simulink model "PubIfDecisionTOS_MDL"  (R2020b)
settings: configuration reference "DspaceConfig" (kept outside this file)
PostLoadFcn:
  | if any(exist('dsrtsu_mdlpostloadfcn', 'file') ~= 0), dsrtsu_mdlpostloadfcn('Execute', bdroot); end
InitFcn:
  | , if any(exist('dsmpb_private', 'file') ~= 0), dsmpb_private('dsmpb_mdlclblib', 'Init', bdroot); end,
undefined symbols (not defined in the file or in its folder): C_TOS_ACCEgoRAxletoFbumplength_m, C_TOS_ACCTargetFront_Flag, C_TOS_AEBJAPedObjDxThre_Val, C_TOS_AEBJAPedObjDyThre_Val, C_TOS_AEBJATargetSize_Val, C_TOS_AEBJAVehObjDxThre_Val, C_TOS_AEBJAVehObjDyThre_Val, C_TOS_AEBJuncPedTargetSize_Val, C_TOS_AEBLatObjDxThre_Val, C_TOS_AEBLatPedDyThre_Val, C_TOS_AEBLatTargetSize_Val, C_TOS_AEBLongTargetInEgoFront_Flag, C_TOS_axAbsGround_Parameter, C_TOS_CameraConfirmedFlag, C_TOS_CNsubjWidth, C_TOS_CurrentLaneCoreMinWidth_Val, C_TOS_CutInProb_Val_Zero, C_TOS_CutOutProb_Val_Zero, C_TOS_D2R_Val, C_TOS_DefaultValueObjectToCenterLine_dy, C_TOS_EgoCarWidth_Val, C_TOS_EgoDxRefPoint_m, C_TOS_EgoRAxletoFbumplength_m, C_TOS_HalfWidthVehicle_Con, C_TOS_HWA_CurrentLaneFlag, C_TOS_HWA_LeftLaneFlag, C_TOS_HWA_MovingDir_Vaild, C_TOS_HWA_MovState_Vaild, C_TOS_HWA_RightLaneFlag, C_TOS_LaneLineCourseErrorFront, C_TOS_LaneLineCourseErrorRear, C_TOS_MotorbikeDefaultWidth_m, C_TOS_NumberOfEffectiveTargets, C_TOS_Obj_Age_Val, C_TOS_Objdx_Constraint_Val, C_TOS_ObjectDefaultWidth_m, C_TOS_ObjInCurrentLane_Val, C_TOS_ObjInCurrentLaneValid, C_TOS_ObjInLeftLaneValid, C_TOS_ObjInRightLaneValid, C_TOS_ObjNotInCurrentLane_Val, C_TOS_ObjNotREElementType, C_TOS_ObjPredictDis_dy_ConstantVal_Zeros, C_TOS_ObjToCenterLine_ConstantVal_Zeros, C_TOS_OFMObjIDInvilad_Val, C_TOS_PIL_LatDisCons_Val_zero, C_TOS_PIL_ObjectCutInFlag_b, C_TOS_PIL_ObjectCutOutFlag_b, C_TOS_PIL_ObjLaneProb_al_Val, C_TOS_PP_ObjFusType_FC_Confirm_b, C_TOS_PP_ObjFusType_FC_FR_Confirm_b, C_TOS_PP_ObjFusType_FR_Confirm_b, C_TOS_RE_80BoolDefault_Val, C_TOS_RE_80Single181Default_Val, C_TOS_RE_80Single255Default_Val, C_TOS_RE_80Uint8Default_Val, C_TOS_RE_D2R, C_TOS_RE_D_180_Val, C_TOS_RE_InvalidObjectID_Val, C_TOS_RE_InvalidTargetChainDir_Val ... (+142)
libraries: simulink x1650, TOS_LIB x361, canfdmsglib x14
(part 54 of 69)

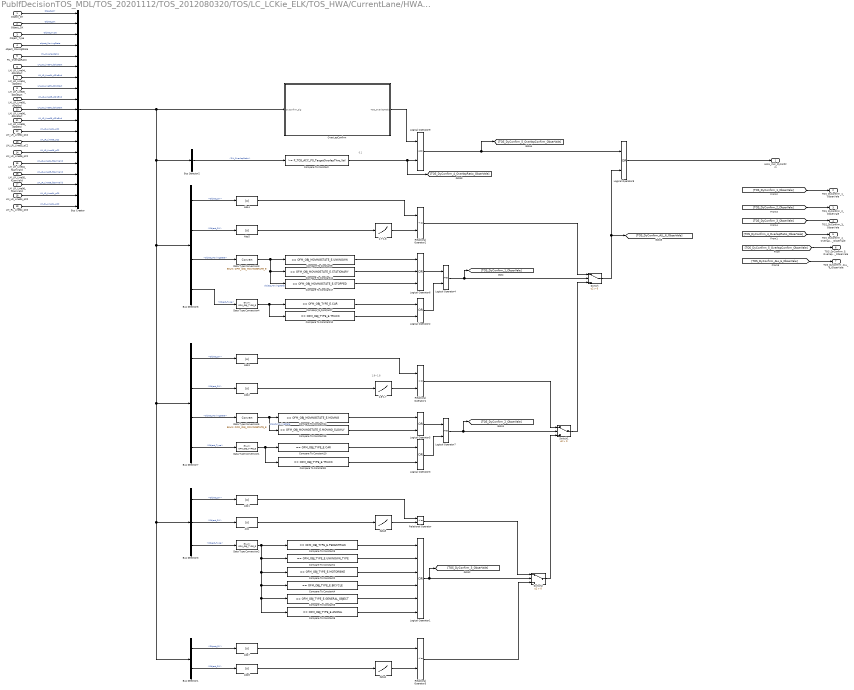
== system PubIfDecisionTOS_MDL/TOS_20201112/TOS_2012080320/TOS/LC_LCKie_ELK/TOS_HWA/CurrentLane/HWA_CurrentLane_Target/HWA_CLF_Target_1/HWA_CLF_Target/HWA_CLF_Target/HWA_CLF_DyConfirm ==
  note: 0.1
  note: 1.9~1.8
  Object_DY : Inport
  Object_DX : Inport  Port=2
  Object_Type : Inport  Port=3
  object_MovingState : Inport  Port=4
  PIL_OverlapRatio : Inport  Port=5
  LM_LR_Line04_dDisStart : Inport  Port=6
  LM_LR_Line04_dDisEnd : Inport  Port=7
  LM_LR_Line05_dDisStart : Inport  Port=8
  LM_LR_Line05_dDisEnd : Inport  Port=9
  LM_LR_Line06_dDisStart : Inport  Port=10
  LM_LR_Line06_dDisEnd : Inport  Port=11
  LM_LR_Line04_pC2 : Inport  Port=12
  LM_LR_Line05_pC2 : Inport  Port=13
  LM_LR_Line06_pC2 : Inport  Port=14
  LM_LR_Line04_fCamValid : Inport  Port=15
  LM_LR_Line05_fCamValid : Inport  Port=16
  LM_LR_Line06_fCamValid : Inport  Port=17
  LM_LR_Line04_pC0 : Inport  Port=18
  LM_RL_Line04_pC0 : Inport  Port=19
  1.7-1.6 : Lookup_n-D  NumberOfTableDimensions=1  BreakpointsForDimension1=[0,20,40,60,80,100,120,140]  Table=[1.7,1.7,1.65,1.65,1.6,1.6,1.6,1.6]  RndMeth=Simplest  InputSameDT=on
  1.8-1.7 : Lookup_n-D  NumberOfTableDimensions=1  BreakpointsForDimension1=[0,20,40,60,80,100,120,140]  Table=[1.8,1.8,1.75,1.75,1.7,1.7,1.7,1.7]  RndMeth=Simplest  InputSameDT=on
  Abs{,1..7} (8 alike) : Abs
  Bus Creator : BusCreator  Inputs=19
  Bus Selector1 : BusSelector  OutputSignals=Object_DY,Object_DX
  Bus Selector2 : BusSelector  OutputSignals=PIL_OverlapRatio
  Bus Selector3 : BusSelector  OutputSignals=Object_DY,Object_DX,Object_Type
  Bus Selector6 : BusSelector  OutputSignals=Object_DY,Object_DX,object_MovingState,Object_Type
  Bus Selector7 : BusSelector  OutputSignals=Object_DY,Object_DX,object_MovingState,Object_Type
  Compare To Constant : simulink/Logic and Bit Operations/Compare To Constant  relop=>=  const=P_TOS_ACC_P0_TargetOverlapThre_Val  OutDataTypeStr=boolean
      settings: AttributesFormatString=P_TOS_ACC_P0_TargetOverlapThre_Val = 0.3
  Compare To Constant1 : simulink/Logic and Bit Operations/Compare To Constant  relop===  const=OFM_OBJ_TYPE_E.UNKNOWN_TYPE  OutDataTypeStr=boolean
      settings: AttributesFormatString=OFM_OBJ_TYPE_E.UNKNOWN_TYPE = 1
  Compare To Constant10 : simulink/Logic and Bit Operations/Compare To Constant  relop===  const=OFM_OBJ_TYPE_E.CAR  OutDataTypeStr=boolean
      settings: AttributesFormatString=OFM_OBJ_TYPE_E.CAR = 2
  Compare To Constant11 : simulink/Logic and Bit Operations/Compare To Constant  relop===  const=OFM_OBJ_MOVINGSTATE_E.STATIONARY  OutDataTypeStr=boolean
      settings: AttributesFormatString=OFM_OBJ_MOVINGSTATE_E.UNKNOWN = 3
  Compare To Constant12 : simulink/Logic and Bit Operations/Compare To Constant  relop===  const=OFM_OBJ_TYPE_E.TRUCK  OutDataTypeStr=boolean
      settings: AttributesFormatString=OFM_OBJ_TYPE_E.TRUCK = 3
  Compare To Constant14 : simulink/Logic and Bit Operations/Compare To Constant  relop===  const=OFM_OBJ_MOVINGSTATE_E.MOVING  OutDataTypeStr=boolean
      settings: AttributesFormatString=OFM_OBJ_MOVINGSTATE_E.MOVING = 2
  Compare To Constant15 : simulink/Logic and Bit Operations/Compare To Constant  relop===  const=OFM_OBJ_MOVINGSTATE_E.MOVING_SLOWLY  OutDataTypeStr=boolean
      settings: AttributesFormatString=OFM_OBJ_MOVINGSTATE_E.MOVING_SLOWLY = 5
  Compare To Constant17 : simulink/Logic and Bit Operations/Compare To Constant  relop===  const=OFM_OBJ_MOVINGSTATE_E.STOPPED  OutDataTypeStr=boolean
      settings: AttributesFormatString=OFM_OBJ_MOVINGSTATE_E.STOPPED = 4
  Compare To Constant2 : simulink/Logic and Bit Operations/Compare To Constant  relop===  const=OFM_OBJ_TYPE_E.MOTORBIKE  OutDataTypeStr=boolean
      settings: AttributesFormatString=OFM_OBJ_TYPE_E.MOTORBIKE = 4
  Compare To Constant3 : simulink/Logic and Bit Operations/Compare To Constant  relop===  const=OFM_OBJ_TYPE_E.PEDESTRIAN  OutDataTypeStr=boolean
      settings: AttributesFormatString=OFM_OBJ_TYPE_E.PEDESTRIAN = 6
  Compare To Constant4 : simulink/Logic and Bit Operations/Compare To Constant  relop===  const=OFM_OBJ_TYPE_E.BICYCLE  OutDataTypeStr=boolean
      settings: AttributesFormatString=OFM_OBJ_TYPE_E.BICYCLE = 5
  Compare To Constant5 : simulink/Logic and Bit Operations/Compare To Constant  relop===  const=OFM_OBJ_TYPE_E.GENERAL_OBJECT  OutDataTypeStr=boolean
      settings: AttributesFormatString=OFM_OBJ_TYPE_E.GENERAL_OBJECT = 7
  Compare To Constant6 : simulink/Logic and Bit Operations/Compare To Constant  relop===  const=OFM_OBJ_TYPE_E.ANIMAL  OutDataTypeStr=boolean
      settings: AttributesFormatString=OFM_OBJ_TYPE_E.ANIMAL = 8
  Compare To Constant7 : simulink/Logic and Bit Operations/Compare To Constant  relop===  const=OFM_OBJ_TYPE_E.CAR  OutDataTypeStr=boolean
      settings: AttributesFormatString=OFM_OBJ_TYPE_E.CAR = 2
  Compare To Constant8 : simulink/Logic and Bit Operations/Compare To Constant  relop===  const=OFM_OBJ_TYPE_E.TRUCK  OutDataTypeStr=boolean
      settings: AttributesFormatString=OFM_OBJ_TYPE_E.TRUCK = 3
  Compare To Constant9 : simulink/Logic and Bit Operations/Compare To Constant  relop===  const=OFM_OBJ_MOVINGSTATE_E.UNKNOWN  OutDataTypeStr=boolean
      settings: AttributesFormatString=OFM_OBJ_MOVINGSTATE_E.UNKNOWN = 1
  Data Type Conversion1 : DataTypeConversion  OutDataTypeStr=Enum: OFM_OBJ_TYPE_E
  Data Type Conversion2 : DataTypeConversion  OutDataTypeStr=Enum: OFM_OBJ_TYPE_E
  Data Type Conversion3 : DataTypeConversion  OutDataTypeStr=Enum: OFM_OBJ_MOVINGSTATE_E
  Data Type Conversion4 : DataTypeConversion  OutDataTypeStr=Enum: OFM_OBJ_TYPE_E
  Data Type Conversion5 : DataTypeConversion  OutDataTypeStr=Enum: OFM_OBJ_MOVINGSTATE_E
  Logical Operator1 : Logic  Operator=OR  Inputs=6  AllPortsSameDT=off  OutDataTypeStr=boolean
  Logical Operator{2..3,5,8} (4 alike) : Logic  Operator=OR  AllPortsSameDT=off  OutDataTypeStr=boolean
  Logical Operator4 : Logic  AllPortsSameDT=off  OutDataTypeStr=boolean
  Logical Operator6 : Logic  Operator=OR  Inputs=3  AllPortsSameDT=off  OutDataTypeStr=boolean
  Logical Operator7 : Logic  AllPortsSameDT=off  OutDataTypeStr=boolean
  Logical Operator9 : Logic  AllPortsSameDT=off  OutDataTypeStr=boolean
  OverLapConfirm : Subsystem
  Relational Operator{,1..3} (4 alike) : RelationalOperator  Operator=<=  OutDataTypeStr=boolean  RndMeth=Simplest
  Switch : Switch  Criteria=u2 > Threshold
  Switch1 : Switch  Criteria=u2 > Threshold
  Switch2 : Switch  Criteria=u2 > Threshold
  data3 : Lookup_n-D  NumberOfTableDimensions=1  BreakpointsForDimension1=[0,20,40,60,80,100,120,140]  Table=[1.4,1.4,1.3,1.3,1.2,1.2,1.2,1.2]  RndMeth=Simplest  InputSameDT=on
  data4 : Lookup_n-D  NumberOfTableDimensions=1  BreakpointsForDimension1=[0,20,40,60,80,100,120,140]  Table=[1.4,1.4,1.3,1.3,1.2,1.2,1.2,1.2]  RndMeth=Simplest  InputSameDT=on
  HWA_CLF_DyConfirm : Outport
  TOS_DyConfirm_1_ObserVale : Outport  Port=2
  TOS_DyConfirm_2_ObserVale : Outport  Port=3
  TOS_DyConfirm_3_ObserVale : Outport  Port=4
  TOS_DyConfirm_4_OverlapRatio_ObserVale : Outport  Port=5
  TOS_DyConfirm_5_OverlapConfirm_ObserVale : Outport  Port=6
  TOS_DyConfirm_ALL_6_ObserVale : Outport  Port=7
  wires:
  LM_RL_Line04_pC0/1 -> Bus Creator/19  "LM_RL_Line04_pC0"
  LM_LR_Line04_pC0/1 -> Bus Creator/18  "LM_LR_Line04_pC0"
  [TOS_DyConfirm_ALL_6_ObserVale] -> TOS_DyConfirm_ALL_6_ObserVale/1
  [TOS_DyConfirm_5_OverlapConfirm_ObserVale] -> TOS_DyConfirm_5_OverlapConfirm_ObserVale/1
  Compare To Constant/1 -> Logical Operator9/2, [TOS_DyConfirm_4_OverlapRatio_ObserVale]
  OverLapConfirm/1(TOS_OverlapRatio) -> Logical Operator9/1
  Bus Creator/1 -> OverLapConfirm/1(DyConfirm_Sig), Bus Selector2/1, Bus Selector6/1, Bus Selector7/1, Bus Selector3/1, Bus Selector1/1
  LM_LR_Line06_fCamValid/1 -> Bus Creator/17  "LM_LR_Line06_fCamValid"
  LM_LR_Line05_fCamValid/1 -> Bus Creator/16  "LM_LR_Line05_fCamValid"
  LM_LR_Line04_fCamValid/1 -> Bus Creator/15  "LM_LR_Line04_fCamValid"
  LM_LR_Line06_dDisEnd/1 -> Bus Creator/11  "LM_LR_Line06_dDisEnd"
  LM_LR_Line06_pC2/1 -> Bus Creator/14  "LM_LR_Line06_pC2"
  LM_LR_Line06_dDisStart/1 -> Bus Creator/10  "LM_LR_Line06_dDisStart"
  LM_LR_Line04_dDisEnd/1 -> Bus Creator/7  "LM_LR_Line04_dDisEnd"
  LM_LR_Line04_dDisStart/1 -> Bus Creator/6  "LM_LR_Line04_dDisStart"
  LM_LR_Line05_dDisStart/1 -> Bus Creator/8  "LM_LR_Line05_dDisStart"
  LM_LR_Line05_dDisEnd/1 -> Bus Creator/9  "LM_LR_Line05_dDisEnd"
  LM_LR_Line04_pC2/1 -> Bus Creator/12  "LM_LR_Line04_pC2"
  LM_LR_Line05_pC2/1 -> Bus Creator/13  "LM_LR_Line05_pC2"
  [TOS_DyConfirm_4_OverlapRatio_ObserVale] -> TOS_DyConfirm_4_OverlapRatio_ObserVale/1
  Logical Operator8/1 -> HWA_CLF_DyConfirm/1
  Logical Operator9/1 -> Logical Operator8/1, [TOS_DyConfirm_5_OverlapConfirm_ObserVale]
  Bus Selector2/1 -> Compare To Constant/1  "<PIL_OverlapRatio>"
  PIL_OverlapRatio/1 -> Bus Creator/5  "PIL_OverlapRatio"
  Logical Operator7/1 -> Switch1/2, [TOS_DyConfirm_2_ObserVale]
  Logical Operator3/1 -> Logical Operator7/2
  Logical Operator5/1 -> Logical Operator7/1
  Compare To Constant14/1 -> Logical Operator5/1
  Compare To Constant15/1 -> Logical Operator5/2
  Data Type Conversion5/1 -> Compare To Constant14/1, Compare To Constant15/1  "object_MovingState"
  Bus Selector7/3 -> Data Type Conversion5/1  "<object_MovingState>"
  Logical Operator2/1 -> Logical Operator4/2
  Logical Operator6/1 -> Logical Operator4/1
  Compare To Constant17/1 -> Logical Operator6/3
  Compare To Constant11/1 -> Logical Operator6/2
  Compare To Constant9/1 -> Logical Operator6/1
  Bus Selector6/4 -> Data Type Conversion4/1  "<Object_Type>"
  Compare To Constant7/1 -> Logical Operator2/1
  Data Type Conversion4/1 -> Compare To Constant12/1, Compare To Constant7/1
  Compare To Constant12/1 -> Logical Operator2/2
  Data Type Conversion3/1 -> Compare To Constant9/1, Compare To Constant11/1, Compare To Constant17/1  "object_MovingState"
  [TOS_DyConfirm_3_ObserVale] -> TOS_DyConfirm_3_ObserVale/1
  [TOS_DyConfirm_2_ObserVale] -> TOS_DyConfirm_2_ObserVale/1
  [TOS_DyConfirm_1_ObserVale] -> TOS_DyConfirm_1_ObserVale/1
  Relational Operator3/1 -> Switch2/3
  Abs7/1 -> Relational Operator3/1
  data4/1 -> Relational Operator3/2
  Abs6/1 -> data4/1
  Bus Selector1/1 -> Abs7/1  "<Object_DY>"
  Bus Selector1/2 -> Abs6/1  "<Object_DX>"
  Switch2/1 -> Switch1/3
  Switch1/1 -> Switch/3
  Relational Operator1/1 -> Switch1/1
  Relational Operator2/1 -> Switch/1
  Logical Operator4/1 -> Switch/2, [TOS_DyConfirm_1_ObserVale]
  Abs4/1 -> Relational Operator2/1
  1.7-1.6/1 -> Relational Operator2/2
  Abs5/1 -> 1.7-1.6/1
  Bus Selector6/2 -> Abs5/1  "<Object_DX>"
  Bus Selector6/1 -> Abs4/1  "<Object_DY>"
  Bus Selector6/3 -> Data Type Conversion3/1  "<object_MovingState>"
  object_MovingState/1 -> Bus Creator/4  "object_MovingState"
  Object_DX/1 -> Bus Creator/2  "Object_DX"
  Object_DY/1 -> Bus Creator/1  "Object_DY"
  Relational Operator/1 -> Switch2/1
  Abs/1 -> data3/1
  data3/1 -> Relational Operator/2
  Abs1/1 -> Relational Operator/1
  Object_Type/1 -> Bus Creator/3  "Object_Type"
  Bus Selector3/3 -> Data Type Conversion2/1  "<Object_Type>"
  Compare To Constant3/1 -> Logical Operator1/1
  Bus Selector3/2 -> Abs/1  "<Object_DX>"
  Bus Selector3/1 -> Abs1/1  "<Object_DY>"
  Data Type Conversion2/1 -> Compare To Constant1/1, Compare To Constant2/1, Compare To Constant4/1, Compare To Constant5/1, Compare To Constant6/1, Compare To Constant3/1
  Compare To Constant1/1 -> Logical Operator1/2
  Compare To Constant2/1 -> Logical Operator1/3
  Compare To Constant4/1 -> Logical Operator1/4
  Compare To Constant5/1 -> Logical Operator1/5
  Compare To Constant6/1 -> Logical Operator1/6
  Logical Operator1/1 -> Switch2/2, [TOS_DyConfirm_3_ObserVale]
  Compare To Constant8/1 -> Logical Operator3/2
  Data Type Conversion1/1 -> Compare To Constant10/1, Compare To Constant8/1
  Bus Selector7/1 -> Abs3/1  "<Object_DY>"
  Bus Selector7/2 -> Abs2/1  "<Object_DX>"
  Compare To Constant10/1 -> Logical Operator3/1
  Bus Selector7/4 -> Data Type Conversion1/1  "<Object_Type>"
  Abs3/1 -> Relational Operator1/1
  1.8-1.7/1 -> Relational Operator1/2
  Abs2/1 -> 1.8-1.7/1
  Switch/1 -> Logical Operator8/2, [TOS_DyConfirm_ALL_6_ObserVale]

== system PubIfDecisionTOS_MDL/TOS_20201112/TOS_2012080320/TOS/LC_LCKie_ELK/TOS_HWA/CurrentLane/HWA_CurrentLane_Target/HWA_CLF_Target_1/HWA_CLF_Target/HWA_CLF_Target/HWA_CLF_FusionTypeConfirm ==
  note: 针对有选中的运动目标，运动状态突变为静止，改变其运动状态为运动
  note: 延时3帧模块
  object_MovingState : Inport
  PP_ObjFusType_FC_FR_Confirm : Inport  Port=2
  PP_ObjFusType_FR_Confirm : Inport  Port=3
  PP_ObjFusType_FC_Confirm : Inport  Port=4
  HWA_CLF_Target_ID_K1 : Inport  Port=5
  HWA_CLF_Target_ID_K2 : Inport  Port=6
  HWA_CLF_Target_MovState_K1 : Inport  Port=7
  HWA_CLF_Target_MovState_K2 : Inport  Port=8
  ObjectID : Inport  Port=9
  Compare To Constant : simulink/Logic and Bit Operations/Compare To Constant  relop===  const=OFM_OBJ_MOVINGSTATE_E.MOVING  OutDataTypeStr=boolean
      settings: AttributesFormatString=OFM_OBJ_MOVINGSTATE_E.MOVING = 2
  Compare To Constant1 : simulink/Logic and Bit Operations/Compare To Constant  relop===  const=OFM_OBJ_MOVINGSTATE_E.MOVING_SLOWLY  OutDataTypeStr=boolean
      settings: AttributesFormatString=OFM_OBJ_MOVINGSTATE_E.MOVING_SLOWLY = 5
  Compare To Constant2 : simulink/Logic and Bit Operations/Compare To Constant  relop===  const=OFM_OBJ_MOVINGSTATE_E.UNKNOWN  OutDataTypeStr=boolean
      settings: AttributesFormatString=OFM_OBJ_MOVINGSTATE_E.UNKNOWN = 1
  Compare To Constant3 : simulink/Logic and Bit Operations/Compare To Constant  relop===  const=OFM_OBJ_MOVINGSTATE_E.STATIONARY  OutDataTypeStr=boolean
      settings: AttributesFormatString=OFM_OBJ_MOVINGSTATE_E.STATIONARY = 3
  Compare To Constant4 : simulink/Logic and Bit Operations/Compare To Constant  relop===  const=OFM_OBJ_MOVINGSTATE_E.STOPPED  OutDataTypeStr=boolean
      settings: AttributesFormatString=OFM_OBJ_MOVINGSTATE_E.STOPPED = 4
  Compare To Constant5 : simulink/Logic and Bit Operations/Compare To Constant  relop===  const=C_TOS_PP_ObjFusType_FC_Confirm_b  OutDataTypeStr=boolean
      settings: AttributesFormatString=C_TOS_PP_ObjFusType_FC_Confirm_b = 1
  Compare To Constant6 : simulink/Logic and Bit Operations/Compare To Constant  relop===  const=C_TOS_PP_ObjFusType_FR_Confirm_b  OutDataTypeStr=boolean
      settings: AttributesFormatString=C_TOS_PP_ObjFusType_FR_Confirm_b = 1
  Compare To Constant7 : simulink/Logic and Bit Operations/Compare To Constant  relop===  const=C_TOS_PP_ObjFusType_FC_Confirm_b  OutDataTypeStr=boolean
      settings: AttributesFormatString=C_TOS_PP_ObjFusType_FC_Confirm_b = 1
  Compare To Constant8 : simulink/Logic and Bit Operations/Compare To Constant  relop===  const=1  OutDataTypeStr=boolean
  Data Type Conversion1 : DataTypeConversion  OutDataTypeStr=Enum: OFM_OBJ_MOVINGSTATE_E
  Logical Operator1 : Logic  AllPortsSameDT=off  OutDataTypeStr=boolean
  Logical Operator15 : Logic  AllPortsSameDT=off  OutDataTypeStr=boolean
  Logical Operator2 : Logic  Operator=OR  Inputs=4  AllPortsSameDT=off  OutDataTypeStr=boolean
  Logical Operator3 : Logic  Operator=OR  AllPortsSameDT=off  OutDataTypeStr=boolean
  Logical Operator4 : Logic  Operator=OR  AllPortsSameDT=off  OutDataTypeStr=boolean
  Logical Operator5 : Logic  Operator=OR  AllPortsSameDT=off  OutDataTypeStr=boolean
  Subsystem1 : Subsystem
  TOS_ACCFusionTypeAborDly : Subsystem
  Terminator : Terminator
  HWA_CLF_FusionType : Outport
  wires:
  Compare To Constant2/1 -> Logical Operator4/2
  Compare To Constant/1 -> Logical Operator2/1
  Data Type Conversion1/1 -> Compare To Constant/1, Compare To Constant1/1, Compare To Constant4/1, Compare To Constant2/1, Compare To Constant3/1, Subsystem1/1(ObjMovState)
  Logical Operator1/1 -> Logical Operator3/2
  Logical Operator2/1 -> Logical Operator15/2
  object_MovingState/1 -> Data Type Conversion1/1
  Logical Operator15/1 -> Logical Operator3/1
  Compare To Constant4/1 -> Logical Operator2/3
  Logical Operator5/1 -> Logical Operator15/1
  Compare To Constant5/1 -> Logical Operator1/1
  Compare To Constant3/1 -> Logical Operator4/1
  Compare To Constant7/1 -> Logical Operator5/1, [PP_ObjFusType_FC_Confirm]
  Compare To Constant1/1 -> Logical Operator2/2
  [PP_ObjFusType_FC_Confirm] -> Compare To Constant5/1
  Logical Operator4/1 -> Logical Operator1/2
  PP_ObjFusType_FC_Confirm/1 -> Compare To Constant7/1
  PP_ObjFusType_FR_Confirm/1 -> Compare To Constant6/1
  Compare To Constant6/1 -> Logical Operator5/2
  HWA_CLF_Target_ID_K1/1 -> Subsystem1/2(HWA_CLF_Target_ID_K1), [HWA_CLF_Target_ID_K1]
  HWA_CLF_Target_ID_K2/1 -> Subsystem1/3(HWA_CLF_Target_ID_K2)
  ObjectID/1 -> [ObjectID], Subsystem1/6(ObjectID)
  Subsystem1/1(TOS_ObjMovStateCfm) -> Compare To Constant8/1
  Compare To Constant8/1 -> Logical Operator2/4
  HWA_CLF_Target_MovState_K2/1 -> Subsystem1/5(HWA_CLF_Target_MovState_K2)
  HWA_CLF_Target_MovState_K1/1 -> Subsystem1/4(HWA_CLF_Target_MovState_K1)
  TOS_ACCFusionTypeAborDly/1(HWA_CLF_FusionTypeFilt) -> HWA_CLF_FusionType/1
  [ObjectID] -> TOS_ACCFusionTypeAborDly/2(ObjectID)
  [HWA_CLF_Target_ID_K1] -> TOS_ACCFusionTypeAborDly/1(HWA_CLF_TargetP0_ID_K1)
  Logical Operator3/1 -> TOS_ACCFusionTypeAborDly/3(TOS_FusionType)
  PP_ObjFusType_FC_FR_Confirm/1 -> Terminator/1

== system PubIfDecisionTOS_MDL/TOS_20201112/TOS_2012080320/TOS/LC_LCKie_ELK/TOS_HWA/CurrentLane/HWA_CurrentLane_Target/HWA_CLF_Target_1/HWA_CLF_Target/HWA_CLF_Target/HWA_CLF_ObjTypeConfirm ==
  note: 针对有选中的运动目标，运动状态突变为静止，改变其运动状态为运动
  object_MovingState : Inport
  Object_Type : Inport  Port=2
  Target_ID_K1 : Inport  Port=3
  Target_ID_K2 : Inport  Port=4
  Target_MovState_K1 : Inport  Port=5
  Target_MovState_K2 : Inport  Port=6
  ObjectID : Inport  Port=7
  Compare To Constant : simulink/Logic and Bit Operations/Compare To Constant  relop===  const=OFM_OBJ_TYPE_E.CAR  OutDataTypeStr=boolean
      settings: AttributesFormatString=OFM_OBJ_TYPE_E.CAR = 2
  Compare To Constant1 : simulink/Logic and Bit Operations/Compare To Constant  relop===  const=OFM_OBJ_TYPE_E.TRUCK  OutDataTypeStr=boolean
      settings: AttributesFormatString=OFM_OBJ_TYPE_E.TRUCK = 3
  Compare To Constant11 : simulink/Logic and Bit Operations/Compare To Constant  relop===  const=1  OutDataTypeStr=boolean
  Compare To Constant2 : simulink/Logic and Bit Operations/Compare To Constant  relop===  const=OFM_OBJ_MOVINGSTATE_E.MOVING  OutDataTypeStr=boolean
      settings: AttributesFormatString=OFM_OBJ_MOVINGSTATE_E.MOVING = 2
  Compare To Constant3 : simulink/Logic and Bit Operations/Compare To Constant  relop===  const=OFM_OBJ_MOVINGSTATE_E.MOVING_SLOWLY  OutDataTypeStr=boolean
      settings: AttributesFormatString=OFM_OBJ_MOVINGSTATE_E.MOVING_SLOWLY = 5
  Compare To Constant4 : simulink/Logic and Bit Operations/Compare To Constant  relop===  const=OFM_OBJ_TYPE_E.MOTORBIKE  OutDataTypeStr=boolean
      settings: AttributesFormatString=OFM_OBJ_TYPE_E.MOTORBIKE = 4
  Compare To Constant5 : simulink/Logic and Bit Operations/Compare To Constant  relop===  const=OFM_OBJ_TYPE_E.BICYCLE  OutDataTypeStr=boolean
      settings: AttributesFormatString=OFM_OBJ_TYPE_E.BICYCLE = 5
  Compare To Constant6 : simulink/Logic and Bit Operations/Compare To Constant  relop===  const=OFM_OBJ_MOVINGSTATE_E.STOPPED  OutDataTypeStr=boolean
      settings: AttributesFormatString=OFM_OBJ_MOVINGSTATE_E.STOPPED = 4
  Compare To Constant7 : simulink/Logic and Bit Operations/Compare To Constant  relop===  const=OFM_OBJ_TYPE_E.PEDESTRIAN  OutDataTypeStr=boolean
      settings: AttributesFormatString=OFM_OBJ_TYPE_E.PEDESTRIAN = 6
  Compare To Constant8 : simulink/Logic and Bit Operations/Compare To Constant  relop===  const=OFM_OBJ_TYPE_E.UNKNOWN_TYPE  OutDataTypeStr=boolean
      settings: AttributesFormatString=OFM_OBJ_TYPE_E.UNKNOWN_TYPE = 1
  Data Type Conversion : DataTypeConversion  OutDataTypeStr=Enum: OFM_OBJ_TYPE_E
  Data Type Conversion2 : DataTypeConversion  OutDataTypeStr=Enum: OFM_OBJ_MOVINGSTATE_E
  Logical Operator : Logic  AllPortsSameDT=off  OutDataTypeStr=boolean
  Logical Operator1 : Logic  Operator=OR  Inputs=6  AllPortsSameDT=off  OutDataTypeStr=boolean
  Logical Operator2 : Logic  Operator=OR  Inputs=4  AllPortsSameDT=off  OutDataTypeStr=boolean
  Subsystem : Subsystem
  TOS_ObjTypeAborDly : Subsystem
  HWA_CLF_ObjType : Outport
  wires:
  Compare To Constant7/1 -> Logical Operator1/6
  Data Type Conversion2/1 -> Compare To Constant2/1, Compare To Constant3/1, Compare To Constant6/1, Subsystem/1(ObjMovState)
  Target_ID_K1/1 -> Subsystem/2(Target_ID_K1), [Target_ID_K1]
  Target_MovState_K2/1 -> Subsystem/5(Target_MovState_K2)
  Compare To Constant11/1 -> Logical Operator2/4
  Target_MovState_K1/1 -> Subsystem/4(Target_MovState_K1)
  Target_ID_K2/1 -> Subsystem/3(Target_ID_K2)
  Subsystem/1(TOS_ObjMovStateCfm) -> Compare To Constant11/1
  ObjectID/1 -> [ObjectID], Subsystem/6(ObjectID)
  TOS_ObjTypeAborDly/1(ObjTypeFilt) -> HWA_CLF_ObjType/1
  [ObjectID] -> TOS_ObjTypeAborDly/2(ObjectID)
  [Target_ID_K1] -> TOS_ObjTypeAborDly/1(Target_ID_K1)
  Compare To Constant8/1 -> Logical Operator/2
  Logical Operator2/1 -> Logical Operator/1
  Logical Operator1/1 -> TOS_ObjTypeAborDly/3(ObjType)
  Compare To Constant5/1 -> Logical Operator1/5
  Compare To Constant4/1 -> Logical Operator1/4
  Compare To Constant1/1 -> Logical Operator1/3
  Compare To Constant/1 -> Logical Operator1/2
  Logical Operator/1 -> Logical Operator1/1
  object_MovingState/1 -> Data Type Conversion2/1
  Compare To Constant6/1 -> Logical Operator2/3
  Compare To Constant2/1 -> Logical Operator2/1
  Compare To Constant3/1 -> Logical Operator2/2
  Data Type Conversion/1 -> Compare To Constant8/1, Compare To Constant/1, Compare To Constant1/1, Compare To Constant4/1, Compare To Constant5/1, Compare To Constant7/1
  Object_Type/1 -> Data Type Conversion/1

== system PubIfDecisionTOS_MDL/TOS_20201112/TOS_2012080320/TOS/LC_LCKie_ELK/TOS_HWA/CurrentLane/HWA_CurrentLane_Target/HWA_CLF_Target_1/HWA_CLF_Target/HWA_CLF_Target/HWA_CLF_ObstacleProbConfirm ==
  note: 参考值：Prob=0.45
  Target_ID_K1 : Inport
  ObjectID : Inport  Port=2
  Object_ObstacleProb : Inport  Port=3
  Compare To Constant : simulink/Logic and Bit Operations/Compare To Constant  relop=>=  const=P_TOS_ACC_P0_ObstacleProbThre_Valu  OutDataTypeStr=boolean
      settings: AttributesFormatString=P_TOS_ACC_P0_ObstacleProbThre_Valu = 0.4
  ObstacleProbAborDly : Subsystem
  HWA_CLF_ObstacleProb : Outport
  wires:
  ObjectID/1 -> ObstacleProbAborDly/2(ObjectID)
  Target_ID_K1/1 -> ObstacleProbAborDly/1(Target_ID_K1)
  ObstacleProbAborDly/1(ObstacleProbFilt) -> HWA_CLF_ObstacleProb/1
  Compare To Constant/1 -> ObstacleProbAborDly/3(ObstacleProb)
  Object_ObstacleProb/1 -> Compare To Constant/1

== system PubIfDecisionTOS_MDL/TOS_20201112/TOS_2012080320/TOS/LC_LCKie_ELK/TOS_HWA/CurrentLane/HWA_CurrentLane_Target/HWA_CLF_Target_1/HWA_CLF_Target/HWA_CLF_Target/HWA_CLF_TargetDxConfirm ==
  Object_Dx : Inport
  TOS_TLJ_SameLaneConfirm_Flag : Inport  Port=2
  object_MovingState : Inport  Port=3
  Compare To Constant1 : simulink/Logic and Bit Operations/Compare To Constant  relop=<  const=P_TOS_EgoFrontDxThre_120_Val  OutDataTypeStr=boolean
      settings: AttributesFormatString=P_TOS_EgoFrontDxThre_120_Val = 120
  Compare To Constant11 : simulink/Logic and Bit Operations/Compare To Constant  relop===  const=OFM_OBJ_MOVINGSTATE_E.STATIONARY  OutDataTypeStr=boolean
      settings: AttributesFormatString=OFM_OBJ_MOVINGSTATE_E.UNKNOWN = 3
  Compare To Constant2 : simulink/Logic and Bit Operations/Compare To Constant  relop===  const=OFM_OBJ_MOVINGSTATE_E.MOVING  OutDataTypeStr=boolean
      settings: AttributesFormatString=OFM_OBJ_MOVINGSTATE_E.MOVING = 2
  Compare To Constant3 : simulink/Logic and Bit Operations/Compare To Constant  relop===  const=OFM_OBJ_MOVINGSTATE_E.MOVING_SLOWLY  OutDataTypeStr=boolean
      settings: AttributesFormatString=OFM_OBJ_MOVINGSTATE_E.MOVING_SLOWLY = 5
  Compare To Constant4 : simulink/Logic and Bit Operations/Compare To Constant  relop=>=  const=P_TOS_RefPoint_dx_m  OutDataTypeStr=boolean
      settings: AttributesFormatString=P_TOS_RefPoint_dx_m = 0
  Compare To Constant5 : simulink/Logic and Bit Operations/Compare To Constant  relop===  const=OFM_OBJ_MOVINGSTATE_E.UNKNOWN  OutDataTypeStr=boolean
      settings: AttributesFormatString=OFM_OBJ_MOVINGSTATE_E.UNKNOWN = 1
  Compare To Constant6 : simulink/Logic and Bit Operations/Compare To Constant  relop===  const=OFM_OBJ_MOVINGSTATE_E.STOPPED  OutDataTypeStr=boolean
      settings: AttributesFormatString=OFM_OBJ_MOVINGSTATE_E.STOPPED = 4
  Compare To Constant8 : simulink/Logic and Bit Operations/Compare To Constant  relop=<  const=P_TOS_EgoFrontDxThre_90_Val  OutDataTypeStr=boolean
      settings: AttributesFormatString=P_TOS_EgoFrontDxThre_90_Val = 90
  Compare To Constant9 : simulink/Logic and Bit Operations/Compare To Constant  relop=>=  const=P_TOS_RefPoint_dx_m  OutDataTypeStr=boolean
      settings: AttributesFormatString=P_TOS_RefPoint_dx_m = 0
  Data Type Conversion2 : DataTypeConversion  OutDataTypeStr=Enum: OFM_OBJ_MOVINGSTATE_E
  Logical Operator1 : Logic  Operator=OR  Inputs=4  AllPortsSameDT=off  OutDataTypeStr=boolean
  Logical Operator{2..4,7} (4 alike) : Logic  AllPortsSameDT=off  OutDataTypeStr=boolean
  Logical Operator5 : Logic  Operator=OR  AllPortsSameDT=off  OutDataTypeStr=boolean
  Terminator : Terminator
  HWA_CLF_TargetInEgoFront : Outport
  wires:
  TOS_TLJ_SameLaneConfirm_Flag/1 -> Terminator/1
  Logical Operator5/1 -> HWA_CLF_TargetInEgoFront/1
  Logical Operator7/1 -> Logical Operator5/2
  Logical Operator4/1 -> Logical Operator7/2
  Compare To Constant11/1 -> Logical Operator7/1
  Object_Dx/1 -> Compare To Constant4/1, Compare To Constant1/1, Compare To Constant8/1, Compare To Constant9/1
  Compare To Constant9/1 -> Logical Operator4/1
  Compare To Constant8/1 -> Logical Operator4/2
  Compare To Constant5/1 -> Logical Operator1/1
  Logical Operator2/1 -> Logical Operator5/1
  Logical Operator3/1 -> Logical Operator2/2
  Compare To Constant1/1 -> Logical Operator3/2
  Compare To Constant4/1 -> Logical Operator3/1
  Logical Operator1/1 -> Logical Operator2/1
  Compare To Constant6/1 -> Logical Operator1/4
  Compare To Constant3/1 -> Logical Operator1/3
  Compare To Constant2/1 -> Logical Operator1/2
  object_MovingState/1 -> Data Type Conversion2/1
  Data Type Conversion2/1 -> Compare To Constant5/1, Compare To Constant11/1, Compare To Constant6/1, Compare To Constant3/1, Compare To Constant2/1

== system PubIfDecisionTOS_MDL/TOS_20201112/TOS_2012080320/TOS/LC_LCKie_ELK/TOS_HWA/CurrentLane/HWA_CurrentLane_Target/HWA_CLF_Target_1/HWA_CLF_Target/HWA_CLF_Target/HWA_CLF_TargetMovingDirConfirm ==
  note: 已选中目标，前两个周期为运动，
      | 以后为运动，前两个周期为Stopped，以后为Stopped
  note: 约束：横穿目标
  object_MovingState : Inport
  PP_ObjMovingDirSignalProcessing : Inport  Port=2
  Object_HeadingAngle : Inport  Port=3
  Object_VX : Inport  Port=4
  Object_VY : Inport  Port=5
  VIE_EgoVelocity : Inport  Port=6
  SteerWheelAng : Inport  Port=7
  HWA_CLF_Target_ID_K1 : Inport  Port=8
  HWA_CLF_Target_ID_K2 : Inport  Port=9
  HWA_CLF_Target_MovState_K1 : Inport  Port=10
  HWA_CLF_Target_MovState_K2 : Inport  Port=11
  ObjectID : Inport  Port=12
  Object_Type : Inport  Port=13
  Abs : Abs
  Abs1 : Abs
  Abs2 : Abs
  Add : Sum
  Bus Creator : BusCreator  Inputs=13
  Bus Selector : BusSelector  OutputSignals=PP_ObjMovingDirSignalProcessing,Object_VX,VIE_EgoVelocity,Object_VY
  Bus Selector1 : BusSelector  OutputSignals=object_MovingState,HWA_CLF_Target_ID_K1,HWA_CLF_Target_ID_K2,HWA_CLF_Target_MovState_K1,HWA_CLF_Target_MovState_K2,ObjectID,object_MovingState
  Bus Selector2 : BusSelector  OutputSignals=object_MovingState
  Bus Selector3 : BusSelector  OutputSignals=PP_ObjMovingDirSignalProcessing,Object_HeadingAngle
  Bus Selector4 : BusSelector  OutputSignals=Object_Type
  Compare To Constant : simulink/Logic and Bit Operations/Compare To Constant  relop===  const=ObjectMovingOrientation_E.SameDir  OutDataTypeStr=boolean
      settings: AttributesFormatString=ObjectMovingOrientation_E.SameDir = 1
  Compare To Constant1 : simulink/Logic and Bit Operations/Compare To Constant  relop===  const=OFM_OBJ_MOVINGSTATE_E.MOVING  OutDataTypeStr=boolean
      settings: AttributesFormatString=OFM_OBJ_MOVINGSTATE_E.MOVING = 2
  Compare To Constant10 : simulink/Logic and Bit Operations/Compare To Constant  relop=<=  const=P_TOS_ObjLatCroYawAngMaxThre_Val  OutDataTypeStr=boolean
      settings: AttributesFormatString=P_TOS_ObjLatCroYawAngMaxThre_Val = 135
  Compare To Constant11 : simulink/Logic and Bit Operations/Compare To Constant  relop===  const=1  OutDataTypeStr=boolean
  Compare To Constant12 : simulink/Logic and Bit Operations/Compare To Constant  relop===  const=2  OutDataTypeStr=boolean
  Compare To Constant13 : simulink/Logic and Bit Operations/Compare To Constant  relop=<  const=1.5  OutDataTypeStr=boolean
      settings: AttributesFormatString=1.5 m/s
  Compare To Constant14 : simulink/Logic and Bit Operations/Compare To Constant  relop===  const=OFM_OBJ_TYPE_E.PEDESTRIAN  OutDataTypeStr=boolean
      settings: AttributesFormatString=OFM_OBJ_TYPE_E.PEDESTRIAN = 6
  Compare To Constant2 : simulink/Logic and Bit Operations/Compare To Constant  Commented=on  relop=>=  const=P_TOS_ObjInSameDirYawAngMinThre_Val  OutDataTypeStr=boolean
      settings: AttributesFormatString=P_TOS_ObjInSameDirYawAngMinThre_Val = 0
  Compare To Constant3 : simulink/Logic and Bit Operations/Compare To Constant  Commented=on  relop=<=  const=P_TOS_ObjInSameDirYawAngMaxThre_Val  OutDataTypeStr=boolean
      settings: AttributesFormatString=P_TOS_ObjInSameDirYawAngMaxThre_Val = 45
  Compare To Constant4 : simulink/Logic and Bit Operations/Compare To Constant  relop===  const=OFM_OBJ_MOVINGSTATE_E.MOVING_SLOWLY  OutDataTypeStr=boolean
      settings: AttributesFormatString=OFM_OBJ_MOVINGSTATE_E.MOVING_SLOWLY = 5
  Compare To Constant5 : simulink/Logic and Bit Operations/Compare To Constant  relop=<  const=P_TOS_SameDirVyOffset_Val  OutDataTypeStr=boolean
      settings: AttributesFormatString=P_TOS_SameDirVyOffset_Val = 2
  Compare To Constant6 : simulink/Logic and Bit Operations/Compare To Constant  relop===  const=ObjectMovingOrientation_E.Crossing  OutDataTypeStr=boolean
      settings: AttributesFormatString=ObjectMovingOrientation_E.Crossing = 3
  Compare To Constant7 : simulink/Logic and Bit Operations/Compare To Constant  relop=>=  const=P_TOS_LongVyThre_Val  OutDataTypeStr=boolean
      settings: AttributesFormatString=P_TOS_LongVyThre_Val = 2
  Compare To Constant8 : simulink/Logic and Bit Operations/Compare To Constant  relop===  const=OFM_OBJ_MOVINGSTATE_E.STOPPED  OutDataTypeStr=boolean
      settings: AttributesFormatString=OFM_OBJ_MOVINGSTATE_E.STOPPED = 4
  Compare To Constant9 : simulink/Logic and Bit Operations/Compare To Constant  relop=>=  const=P_TOS_ObjInSameDirYawAngMaxThre_Val  OutDataTypeStr=boolean
      settings: AttributesFormatString=P_TOS_ObjInSameDirYawAngMaxThre_Val = 45
  Constant1 : Constant  Value=P_TOS_SameDirVxvOffset_Val
      settings: AttributesFormatString=P_TOS_AEBLong_SameDirVxvOffset_Val = 1
  Constant2 : Constant  Value=0  OutDataTypeStr=boolean
  Constant3 : Constant  OutDataTypeStr=boolean
  Constant4 : Constant  OutDataTypeStr=boolean
  Data Type Conversion : DataTypeConversion  OutDataTypeStr=Enum: OFM_OBJ_TYPE_E
  Data Type Conversion1 : DataTypeConversion  OutDataTypeStr=Enum: ObjectMovingOrientation_E
  Data Type Conversion2 : DataTypeConversion  OutDataTypeStr=Enum: OFM_OBJ_MOVINGSTATE_E
  Data Type Conversion3 : DataTypeConversion  OutDataTypeStr=Enum: OFM_OBJ_MOVINGSTATE_E
  Data Type Conversion4 : DataTypeConversion  OutDataTypeStr=Enum: OFM_OBJ_MOVINGSTATE_E
  Data Type Conversion5 : DataTypeConversion  OutDataTypeStr=Enum: ObjectMovingOrientation_E
  HWA_MovingDirAborDly : Subsystem
  Logical Operator : Logic  AllPortsSameDT=off  OutDataTypeStr=boolean
  Logical Operator1 : Logic  Operator=OR  AllPortsSameDT=off  OutDataTypeStr=boolean
  Logical Operator2 : Logic  Operator=OR  Inputs=3  AllPortsSameDT=off  OutDataTypeStr=boolean
  Logical Operator3 : Logic  Operator=OR  AllPortsSameDT=off  OutDataTypeStr=boolean
  Logical Operator5 : Logic  Operator=OR  Inputs=3  AllPortsSameDT=off  OutDataTypeStr=boolean
  Logical Operator6 : Logic  AllPortsSameDT=off  OutDataTypeStr=boolean
  Logical Operator7 : Logic  Operator=OR  AllPortsSameDT=off  OutDataTypeStr=boolean
  Logical Operator8 : Logic  AllPortsSameDT=off  OutDataTypeStr=boolean
  Relational Operator : RelationalOperator  Operator=<  OutDataTypeStr=boolean  RndMeth=Simplest
  Subsystem : Subsystem
  Switch : Switch  Criteria=u2 > Threshold
  Switch1 : Switch  Criteria=u2 ~= 0
  Switch2 : Switch  Criteria=u2 ~= 0
  HWA_CLF_TrgMovDir : Outport
  HWA_CLF_TrgMovDirFlag_1_ObserVale : Outport  Port=2
  HWA_CLF_TrgMovDirFlag_2_ObserVale : Outport  Port=3
  HWA_CLF_TrgMovDirFlag_3_ObserVale : Outport  Port=4
  HWA_CLF_TrgMovDirFlag_4_ObserVale : Outport  Port=5
  HWA_CLF_TrgMovDirFlag_5_ObserVale : Outport  Port=6
  HWA_CLF_TrgMovDirFlag_6_ObserVale : Outport  Port=7
  wires:
  Switch/1 -> Logical Operator3/2
  Compare To Constant14/1 -> Logical Operator3/1
  Bus Selector4/1 -> Data Type Conversion/1  "<Object_Type>"
  Data Type Conversion/1 -> Compare To Constant14/1
  Object_Type/1 -> Bus Creator/13  "Object_Type"
  Bus Selector3/1 -> Data Type Conversion5/1  "<PP_ObjMovingDirSignalProcessing>"
  Data Type Conversion4/1 -> Compare To Constant8/1
  Bus Selector1/7 -> Data Type Conversion4/1  "<object_MovingState>"
  Data Type Conversion3/1 -> Subsystem/1(ObjMovState)
  Bus Selector1/1 -> Data Type Conversion3/1  "<object_MovingState>"
  Bus Creator/1 -> Bus Selector4/1, Bus Selector/1, Bus Selector2/1, Bus Selector1/1, Bus Selector3/1
  ObjectID/1 -> Bus Creator/12  "ObjectID"
  HWA_CLF_Target_MovState_K2/1 -> Bus Creator/11  "HWA_CLF_Target_MovState_K2"
  HWA_CLF_Target_MovState_K1/1 -> Bus Creator/10  "HWA_CLF_Target_MovState_K1"
  HWA_CLF_Target_ID_K2/1 -> Bus Creator/9  "HWA_CLF_Target_ID_K2"
  HWA_CLF_Target_ID_K1/1 -> Bus Creator/8  "HWA_CLF_Target_ID_K1"
  VIE_EgoVelocity/1 -> Bus Creator/6  "VIE_EgoVelocity"
  Object_VY/1 -> Bus Creator/5  "Object_VY"
  Object_VX/1 -> Bus Creator/4  "Object_VX"
  Object_HeadingAngle/1 -> Bus Creator/3  "Object_HeadingAngle"
  object_MovingState/1 -> Bus Creator/1  "object_MovingState"
  PP_ObjMovingDirSignalProcessing/1 -> Bus Creator/2  "PP_ObjMovingDirSignalProcessing"
  Compare To Constant13/1 -> Logical Operator8/2
  [Object_VY] -> Compare To Constant13/1
  Constant4/1 -> Logical Operator8/1
  HWA_MovingDirAborDly/2(HWA_TrgMovDir) -> HWA_CLF_TrgMovDir/1
  HWA_MovingDirAborDly/1(HWA_TrgMovDirFlag_6_ObserVale) -> [HWA_CLF_TrgMovDirFlag_6_ObserVale]
  [HWA_CLF_TrgMovDirFlag_6_ObserVale] -> HWA_CLF_TrgMovDirFlag_6_ObserVale/1
  [HWA_CLF_TrgMovDirFlag_5_ObserVale] -> HWA_CLF_TrgMovDirFlag_5_ObserVale/1
  [HWA_CLF_TrgMovDirFlag_4_ObserVale] -> HWA_CLF_TrgMovDirFlag_4_ObserVale/1
  [HWA_CLF_TrgMovDirFlag_3_ObserVale] -> HWA_CLF_TrgMovDirFlag_3_ObserVale/1
  [HWA_CLF_TrgMovDirFlag_2_ObserVale] -> HWA_CLF_TrgMovDirFlag_2_ObserVale/1
  [HWA_CLF_TrgMovDirFlag_1_ObserVale] -> HWA_CLF_TrgMovDirFlag_1_ObserVale/1
  Logical Operator7/1 -> Switch2/2, [HWA_CLF_TrgMovDirFlag_3_ObserVale]
  Compare To Constant12/1 -> Logical Operator7/1
  Bus Selector1/2 -> Subsystem/2(ACC_Target_ID_K1), [HWA_CLF_Target_ID_K1]  "<HWA_CLF_Target_ID_K1>"
  Bus Selector1/4 -> Subsystem/4(ACC_Target_MovState_K1)  "<HWA_CLF_Target_MovState_K1>"
  Bus Selector1/3 -> Subsystem/3(ACC_Target_ID_K2)  "<HWA_CLF_Target_ID_K2>"
  Bus Selector1/5 -> Subsystem/5(ACC_Target_MovState_K2)  "<HWA_CLF_Target_MovState_K2>"
  Data Type Conversion2/1 -> Compare To Constant4/1, Compare To Constant1/1
  Subsystem/1(TOS_ObjMovStateCfm) -> Compare To Constant12/1, Compare To Constant11/1
  Compare To Constant11/1 -> Logical Operator2/3
  Bus Selector1/6 -> Subsystem/6(ObjectID), [ObjectID]  "<ObjectID>"
  Logical Operator8/1 -> Switch2/1
  Switch2/1 -> Switch/3
  Compare To Constant8/1 -> Logical Operator7/2
  Switch1/1 -> Switch2/3
  Logical Operator6/1 -> Logical Operator5/2
  Compare To Constant10/1 -> Logical Operator6/2
  Compare To Constant9/1 -> Logical Operator6/1
  Abs/1 -> Compare To Constant9/1, Compare To Constant10/1
  Compare To Constant6/1 -> Logical Operator5/1
  Data Type Conversion5/1 -> Compare To Constant6/1
  Logical Operator3/1 -> [HWA_CLF_TrgMovDirFlag_5_ObserVale], HWA_MovingDirAborDly/3(HWA_MovingDir)
  [ObjectID] -> HWA_MovingDirAborDly/2(ObjectID)
  [HWA_CLF_Target_ID_K1] -> HWA_MovingDirAborDly/1(HWA_TargetP0_ID_K1)
  [Object_VY] -> Compare To Constant7/1
  Compare To Constant7/1 -> Logical Operator5/3
  Constant2/1 -> Switch1/1
  Logical Operator5/1 -> Switch1/2, [HWA_CLF_TrgMovDirFlag_4_ObserVale]
  Constant3/1 -> Switch1/3
  SteerWheelAng/1 -> Bus Creator/7  "SteerWheelAng"
  Abs2/1 -> [Object_VY], Compare To Constant5/1
  Bus Selector/4 -> Abs2/1  "<Object_VY>"
  Bus Selector/2 -> Abs1/1  "<Object_VX>"
  Bus Selector/3 -> Relational Operator/2  "<VIE_EgoVelocity>"
  Add/1 -> Relational Operator/1
  Constant1/1 -> Add/2
  Abs1/1 -> Add/1
  Relational Operator/1 -> Logical Operator/1
  Compare To Constant5/1 -> Logical Operator/2
  Logical Operator/1 -> Logical Operator1/2
  Bus Selector/1 -> Data Type Conversion1/1  "<PP_ObjMovingDirSignalProcessing>"
  Logical Operator1/1 -> [HWA_CLF_TrgMovDirFlag_1_ObserVale], Switch/1
  Data Type Conversion1/1 -> Compare To Constant/1
  Bus Selector3/2 -> Abs/1  "<Object_HeadingAngle>"
  Compare To Constant/1 -> Logical Operator1/1
  Bus Selector2/1 -> Data Type Conversion2/1  "<object_MovingState>"
  Compare To Constant4/1 -> Logical Operator2/2
  Compare To Constant1/1 -> Logical Operator2/1
  Logical Operator2/1 -> Switch/2, [HWA_CLF_TrgMovDirFlag_2_ObserVale]
